simulink model "BoundingBoxWidthtoHeightRatio"  (R2016a)
settings: Solver=VariableStepAuto  StartTime=0.0  StopTime=inf  RelTol=1e-3
undefined symbols (not defined in the file): none, videoinput
libraries: imaqlib x1, visionsinks x1
settings Model: Creator=YASARA  LastModifiedBy=YASARA

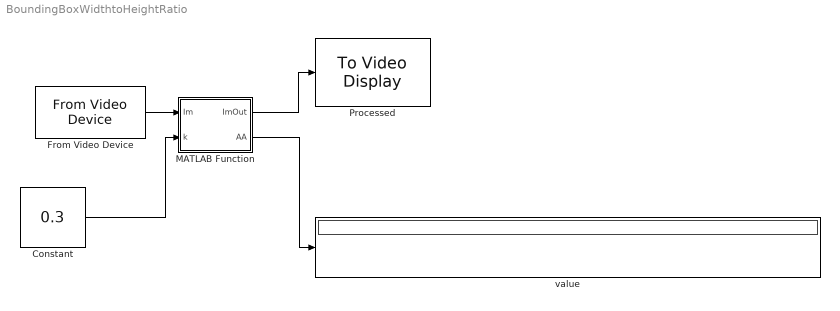
== system BoundingBoxWidthtoHeightRatio ==
  Constant : Constant  Value=0.3  OutDataTypeStr=double  SampleTime=100000
  From Video Device : imaqlib/From Video Device  DeviceMenu=winvideo 2 (USB Video Device)  Device=winvideo 2 (USB Video Device)  ObjConstructor=videoinput('winvideo', 2)  VideoFormatMenu=YUY2_160x120  VideoFormat=YUY2_160x120  VideoSource=input1  ROIPosition=[0 0 120 160]  EnableHWTrigger=off  TriggerConfiguration=none/none  SampleTime=1/30  OutputPortsMode=One multidimensional signal  DataType=double  CanDoHWTrigger=no  ReturnedColorSpace=rgb  BlockHandle=44.0042  ROIWidth=160  ROIHeight=120  ROIColumn=0  ROIRow=0  EngXMLPath=C:\Program Files\MATLAB\R2016a\toolbox\imaq\imaq\private  DevXMLPath=C:\MATLAB\SupportPackages\R2016a\toolbox\imaq\supportpackages\genericvideo\adaptor\win64  EngLibPath=C:\Program Files\MATLAB\R2016a\toolbox\imaq\imaqblks\imaqmex\win64  ColorSpace=rgb  BayerSensorAlignment=grbg
  MATLAB Function : MATLAB Function  TreatAsAtomicUnit=on
  Processed : visionsinks/To Video Display  windowSizeMode=Normal  openAtMdlStart=on  fullScreen=off  videoWindowX=784  videoWindowY=165  saveWindowSize=off  videoWindowWidth=512  videoWindowHeight=384  inputColorFormat=RGB  inputType=Obsolete  imagePorts=One multidimensional signal  OutputDevice=On-screen video monitor  dataOrg=Column-major  isWindowOpen=off
  value : Display
  wires:
  From Video Device/1 -> MATLAB Function/1(Im)
  MATLAB Function/1(ImOut) -> Processed/1
  Constant/1 -> MATLAB Function/2(k)
  MATLAB Function/2(AA) -> value/1

== matlab function BoundingBoxWidthtoHeightRatio/MATLAB Function ==
  data: Im input; ImOut output; k input; AA output
function [ImOut,AA] = fcn(Im,k)
I=rgb2gray(Im);
coder.extrinsic('graythresh');
coder.extrinsic('im2bw');
level = graythresh(I);
BW = im2bw(I,level);
L=double(I);
coder.extrinsic('bwlabeln');
NUM=1;
BW2=imcomplement(BW);
[L, NUM] = bwlabeln(BW2);
area=1;
n=1;
R1=Im(:,:,1);
R2=Im(:,:,2);
R3=Im(:,:,3);
AA=(zeros(50,1));
i=1;
for n=1:NUM
    [r, c] = find(L==n);
    %if (max(c)~= min(c))&&(max(r)~= min(r))
    if ((max(c)-min(c))>5)&&((max(r)-min(r))>5)
        AA(i)=(max(c)-min(c))/(max(r)-min(r));        
        if (AA(i)>k)
           R1(L==n)=0; 
           R2(L==n)=255;            
           R3(L==n)=0;
        end
        i=i+1;
    end
end
II=Im;
II=cat(3,R1,R2,R3);
ImOut=II;
